simulink model "mri_2d_fft_aie_HLS_Kernel"  (R2019b)
settings: Solver=VariableStepAuto  StartTime=0.0  StopTime=256*256*2  RelTol=1e-3
PreLoadFcn:
  | % display k space image & load arrays for
  | % simulation run
  | preload_fcn;
  | 
  | % configure hardware specific information
  | clock_frequency = 150e6;
InitFcn:
  | xmcCheckSlxPath(bdroot);
undefined symbols (not defined in the file or in its folder): gray
libraries: ModelComposer x9, dspsrcs4 x2, xmcCopyrightNotice x1
settings Model: Creator=mmi  LastModifiedBy=abehbood
settings DataIOCC: ReturnWorkspaceOutputs=off
settings DebuggingCC: PregeneratedLibrarySubsystemCodeDiagnostic=none  ArithmeticOperatorsInVariantConditions=warning
settings SFSimCC: SimUseLocalCustomCode=off  CustomCodeUndefinedFunction=UseInterfaceOnly
settings RTWCC: RTWUseLocalCustomCode=off

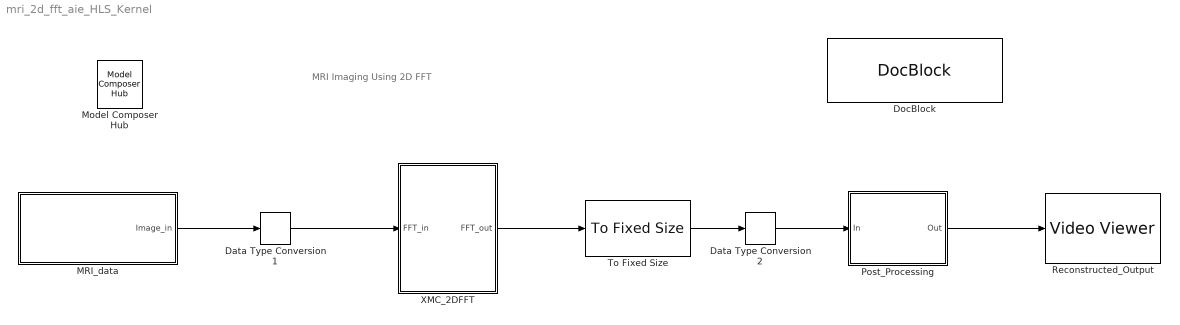
== system mri_2d_fft_aie_HLS_Kernel ==
  note: MRI Imaging Using 2D FFT
  Data Type Conversion1 : ModelComposer/Data Type Conversion  OutDataType=int16  TypeExp=''  Signedness=Signed  WordLength=16  FractionalLength=0  RoundingMode=Truncation to minus infinity  OverflowMode=Wrap around
  Data Type Conversion2 : ModelComposer/Data Type Conversion  OutDataType=int16  TypeExp=''  Signedness=Signed  WordLength=16  FractionalLength=0  RoundingMode=Truncation to minus infinity  OverflowMode=Wrap around
  DocBlock : xmcCopyrightNotice/DocBlock
      content=|
      | (c) Copyright 2017-2018 Xilinx, Inc. All rights reserved.
      |
      | This file contains confidential and proprietary information of Xilinx, Inc.
      | and is protected under U.S. and international copyright and other
      | intellectual property laws.
      |
      | DISCLAIMER
      | This disclaimer is not a license and does not grant any rights to the
      | materials distributed herewith. Except as otherwise provided in a valid
      | license issued to you by Xilinx, and to the maximum extent permitted by
      | applicable law: (1) THESE MATERIALS ARE MADE AVAILABLE "AS IS" AND WITH
      | ALL FAULTS, AND XILINX HEREBY DISCLAIMS ALL WARRANTIES AND CONDITIONS,
      | EXPRESS, IMPLIED, OR STATUTORY, INCLUDING BUT NOT LIMITED TO WARRANTIES
      | OF MERCHANTABILITY, NON-INFRINGEMENT, OR FITNESS FOR ANY PARTICULAR
      | PURPOSE; and (2) Xilinx shall not be liable (whether in contract or tort,
      | including negligence, or under any other theory of liability) for any
      | loss or damage of any kind or nature related to, arising under or in
      | connection with these materials, including for any direct, or any indirect,
      | special, incidental, or consequential loss or damage (including loss of
      | data, profits, goodwill, or any type of loss or damage suffered as a
      | result of any action brought by a third party) even if such damage or loss
      | was reasonably foreseeable or Xilinx had been advised of the possibility
      | of the same.
      |
      | CRITICAL APPLICATIONS
      | Xilinx products are not designed or intended to be fail-safe, or for use
      | in any application requiring fail-safe performance, such as life-support
      | or safety devices or systems, Class III medical devices, nuclear
      | facilities, applications related to the deployment of airbags, or
      | any other applications that could lead to death, personal injury, or
      | severe property or environmental damage (individually and collectively,
      | "Critical Applications"). Customer assumes the sole risk and liability
      | of any use of Xilinx products in Critical Applications, subject only to
      | applicable laws and regulations governing limitations on product liability.
      |
      | THIS COPYRIGHT NOTICE AND DISCLAIMER MUST BE RETAINED AS PART OF
      | THIS FILE AT ALL TIMES.
      settings: SourceProductName=Simulink  SourceProductBaseCode=SL
  MRI_data : Subsystem
  Model Composer Hub : ModelComposer/Model Composer Hub  CodeGeneration=off  TargetDirectory=./code  SubsystemName=XMC_2DFFT  ExportType=IP Catalog  IpVendor=xilinx.com  IpLibrary=hls  IpName=DUT  IpVersion=1.0  IpHWLanguage=Verilog  CreateTestbench=off  TestbenchStackSize=10  AieCompilerOptions={}  RunAieSim=off  LaunchVitisAnalyzer=off  AieSimTimeout=50000  RunX86Sim=on  X86SimTimeout=10  ProjDevice=xcvu11p-flga2577-3-e  ProjDevicePart=xcvu11p-flga2577-3-e  SamplePeriod=-1  ClockFrequency=250  DataPathParallelism=1
  Post_Processing : Subsystem
  Reconstructed_Output : VideoViewer  colormapValue=gray(256)  FigPos=[60 658 635 329]
  To Fixed Size : ModelComposer/To Fixed Size  OutputSize=256  HasStatusOutput=off
  XMC_2DFFT : Subsystem
      mask Display: xmcDrawBlockIcon();
  wires:
  Data Type Conversion1/1 -> XMC_2DFFT/1(FFT_in)
  Data Type Conversion2/1 -> Post_Processing/1(In)
  MRI_data/1(Image_in) -> Data Type Conversion1/1
  Post_Processing/1(Out) -> Reconstructed_Output/1
  To Fixed Size/1 -> Data Type Conversion2/1
  XMC_2DFFT/1(FFT_out) -> To Fixed Size/1

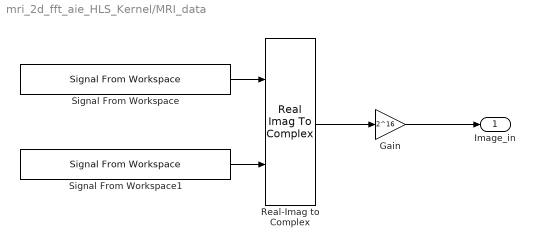
== system mri_2d_fft_aie_HLS_Kernel/MRI_data ==
  Gain : Gain  Gain=2^16
  Real-Imag to Complex : RealImagToComplex
  Signal From Workspace : dspsrcs4/Signal From Workspace  X=MRIDemo_data_real_channel  Ts=1  nsamps=256  OutputAfterFinalValue=Setting to zero  ignoreOrWarnInputAndFrameLengths=off  OutputFrames=off
  Signal From Workspace1 : dspsrcs4/Signal From Workspace  X=MRIDemo_data_imag_channel  Ts=1  nsamps=256  OutputAfterFinalValue=Setting to zero  ignoreOrWarnInputAndFrameLengths=off  OutputFrames=off
  Image_in : Outport  VectorParamsAs1DForOutWhenUnconnected=off
  wires:
  Signal From Workspace/1 -> Real-Imag to Complex/1
  Real-Imag to Complex/1 -> Gain/1
  Signal From Workspace1/1 -> Real-Imag to Complex/2
  Gain/1 -> Image_in/1

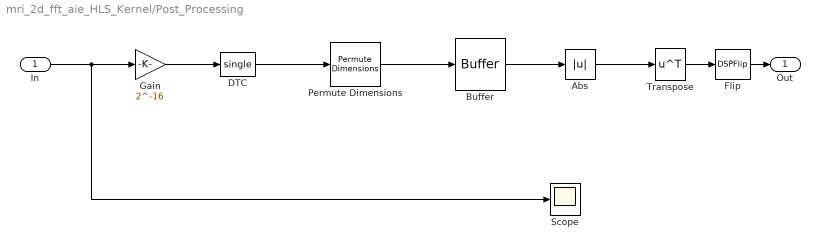
== system mri_2d_fft_aie_HLS_Kernel/Post_Processing ==
  In : Inport
  Abs : Abs
  Buffer : Buffer  N=256  OutputFrames=off
  DTC : DataTypeConversion  OutDataTypeStr=single  RndMeth=Convergent
  Flip : DSPFlip
  Gain : Gain  Gain=2^-16  OutDataTypeStr=fixdt(1,16,15)
  Permute Dimensions : PermuteDimensions
  Scope : Scope
  Transpose : Math  Operator=transpose  SaturateOnIntegerOverflow=on
  Out : Outport  VectorParamsAs1DForOutWhenUnconnected=off
  wires:
  DTC/1 -> Permute Dimensions/1
  Permute Dimensions/1 -> Buffer/1
  Abs/1 -> Transpose/1
  Gain/1 -> DTC/1
  Buffer/1 -> Abs/1
  In/1 -> Scope/1, Gain/1
  Transpose/1 -> Flip/1
  Flip/1 -> Out/1

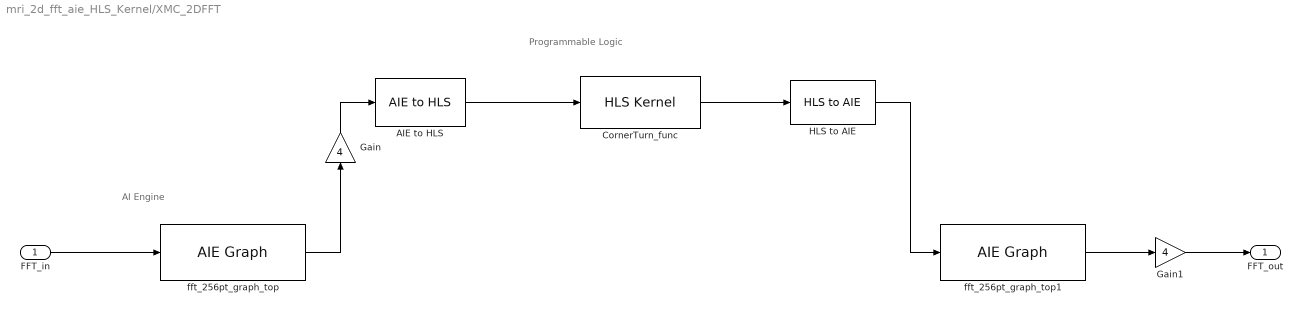
== system mri_2d_fft_aie_HLS_Kernel/XMC_2DFFT ==
  note: Programmable Logic
  note: AI Engine
  FFT_in : Inport
  AIE to HLS : ModelComposer/AIE to HLS  OutputType=ap_axis<64,0,0,0>  OutputSize=128
  CornerTurn_func : ModelComposer/HLS Kernel  PortAttributesTable={'Input', 'in1', 'adf::dir::in< hls::stream< hls::axis< ap_int< 64 >, 0, 0, 0 >, 0 > & >', '', '';'Output', 'out1', 'adf::dir::out< hls::stream< hls::axis< ap_int< 64 >, 0, 0, 0 >, 0 > & >', '', '128'}  PortAttributesEnablement={'off', 'off', 'off', 'off', 'off';'off', 'off', 'off', 'off', 'on'}  FormalArgDecls={'adf::dir::in< hls::stream< hls::axis< ap_int< 64 >, 0, 0, 0 >, 0 > & > in1', 'adf::dir::out< hls::stream< hls::axis< ap_int< 64 >, 0, 0, 0 >, 0 > & > out1'}  PortSynchronicities={'sync', 'sync'}  PortSignalSizes={0.000000000000000000e+00, 1.280000000000000000e+02}  SimLibPath=''  FunctionTabVisible=on  FunctionDescription=void CornerTurn_func(adf::dir::in< hls::stream< hls::axis< ap_int< 64 >, 0, 0, 0 >, 0 > & > in1, adf::dir::out< hls::stream< hls::axis< ap_int< 64 >, 0, 0, 0 >, 0 > & > out1)  KernelHeaderFile=src_corner_turn_hls_kernel/corner_turn_cdno.h  KernelFunction=CornerTurn_func  KernelFunctionSelect=<empty>  KernelSourceFile=src_corner_turn_hls_kernel/corner_turn.cpp  KernelSearchPaths={'./src_corner_turn_hls_kernel'}  PreProcOptions={}
  Gain : Gain  Gain=4  OutDataTypeStr=Inherit: Same as input
  Gain1 : Gain  Gain=4  OutDataTypeStr=Inherit: Same as input
  HLS to AIE : ModelComposer/HLS to AIE  OutputType=cint16  OutputSize=256
  fft_256pt_graph_top : ModelComposer/AIE Graph  PortAttributesTable={'Input', 'in1', 'platform.src[0]', 'top_in', 'window', 'cint16', '256', 'sync', '';'Output', 'out1', 'platform.sink[0]', 'top_out', 'window', 'cint16', '256', 'sync', ''}  PortAttributesEnablement={'off', 'off', 'off', 'on', 'off', 'off', 'off', 'off', 'off';'off', 'off', 'off', 'on', 'off', 'off', 'off', 'off', 'off'}  PortArgDecls={'in window cint16 in1'; 'out window cint16 out1'}  PortNames={'in1'; 'out1'}  PortAliases={'platform.src[0]'; 'platform.sink[0]'}  PortGraphPortNames={'top_in', 'top_out'}  PortTypes={'window'; 'window'}  PortDataTypes={'cint16'; 'cint16'}  PortSizes={2.560000000000000000e+02; 2.560000000000000000e+02}  PortSynchronicities={'sync', 'sync'}  PortSignalSizes={0.000000000000000000e+00, 0.000000000000000000e+00}  SimLibPath=''  FunctionTabVisible=on  GraphName=fft_256pt_graph_top  GraphHeaderFiles={'graph_2d_fft/fft_256pt_graph_top.h'; './fft_256/inc/fft_256pt_graph.h'}  GraphSourceFile=graph_2d_fft/fft_256pt_graph_top.cpp  GraphSearchPaths={'./graph_2d_fft', './fft_256/src', './fft_256/inc'}  GraphPreProcOptions={}
  fft_256pt_graph_top1 : ModelComposer/AIE Graph  PortAttributesTable={'Input', 'in1', 'platform.src[0]', 'top_in', 'window', 'cint16', '256', 'sync', '';'Output', 'out1', 'platform.sink[0]', 'top_out', 'window', 'cint16', '256', 'sync', ''}  PortAttributesEnablement={'off', 'off', 'off', 'on', 'off', 'off', 'off', 'off', 'off';'off', 'off', 'off', 'on', 'off', 'off', 'off', 'off', 'off'}  PortArgDecls={'in window cint16 in1'; 'out window cint16 out1'}  PortNames={'in1'; 'out1'}  PortAliases={'platform.src[0]'; 'platform.sink[0]'}  PortGraphPortNames={'top_in', 'top_out'}  PortTypes={'window'; 'window'}  PortDataTypes={'cint16'; 'cint16'}  PortSizes={2.560000000000000000e+02; 2.560000000000000000e+02}  PortSynchronicities={'sync', 'sync'}  PortSignalSizes={0.000000000000000000e+00, 0.000000000000000000e+00}  SimLibPath=''  FunctionTabVisible=on  GraphName=fft_256pt_graph_top  GraphHeaderFiles={'graph_2d_fft/fft_256pt_graph_top.h'; './fft_256/inc/fft_256pt_graph.h'}  GraphSourceFile=graph_2d_fft/fft_256pt_graph_top.cpp  GraphSearchPaths={'./graph_2d_fft', './fft_256/src', './fft_256/inc'}  GraphPreProcOptions={}
  FFT_out : Outport  VectorParamsAs1DForOutWhenUnconnected=off
  wires:
  fft_256pt_graph_top1/1 -> Gain1/1
  FFT_in/1 -> fft_256pt_graph_top/1
  Gain1/1 -> FFT_out/1
  fft_256pt_graph_top/1 -> Gain/1
  AIE to HLS/1 -> CornerTurn_func/1
  CornerTurn_func/1 -> HLS to AIE/1
  HLS to AIE/1 -> fft_256pt_graph_top1/1
  Gain/1 -> AIE to HLS/1
